simulink model "RPC"  (R2017b)
settings: Solver=FixedStepDiscrete  StartTime=0.0  StopTime=.1  FixedStep=T/100  RelTol=1e-20  AbsTol=1e-20  EnableMultiTasking=on
values from neighbouring files (symbols this model uses):
  n = n(2:3)    [RPC_script.m]
  T = 60/3600/50    (= 0.000333333333333)    [RPC_script.m]    (also in ZPETC_script.m = 0.3)
undefined symbols (not defined in the file or in its folder): d, Wd
libraries: cstblocks x1
settings Model: Creator=oboe  LastModifiedBy=oboe
settings SolverCC: ShapePreserveControl=EnableAll  AutoInsertRateTranBlk=on
settings DataIOCC: LimitDataPoints=on  SaveFormat=Array
settings OptimizationCC: LifeSpan=inf
settings DebuggingCC: SolverPrmCheckMsg=warning  SFUnexpectedBacktrackingDiag=warning  SFNoUnconditionalDefaultTransitionDiag=warning  SFExecutionAtInitializationDiag=none
settings HardwareCC: ProdBitPerPointer=32  ProdBitPerSizeT=32  ProdBitPerPtrDiffT=32  ProdLargestAtomicFloat=None  ProdIntDivRoundTo=Undefined  ProdEndianess=Unspecified  ProdWordSize=32  ProdHWDeviceType=32-bit Generic
settings ModelReferenceCC: PropagateSignalLabelsOutOfModel=off
settings CodeAppCC: StateflowObjectComments=on
settings GRTTargetCC: TargetLangStandard=C89/C90 (ANSI)  GeneratePreprocessorConditionals=Disable all
settings ConfigComp: CovMetricSettings=dw  CovHtmlReporting=on  CovSaveCumulativeToWorkspaceVar=on  CovSaveSingleToWorkspaceVar=on  CovExternalEMLEnable=off  CovSFcnEnable=off

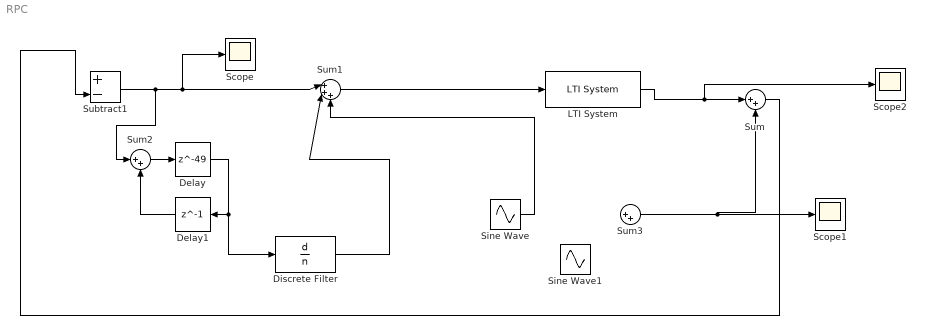
== system RPC ==
  Delay : Delay  DelayLength=49  UseCircularBuffer=on  SampleTime=T
  Delay1 : Delay  DelayLength=1  UseCircularBuffer=on  SampleTime=T
  Discrete Filter : DiscreteFilter  Numerator=d  Denominator=n
  LTI System : cstblocks/LTI System  sys=Wd/(1-Wd)  IC=[]
  Scope : Scope
  Scope1 : Scope
  Scope2 : Scope
  Sine Wave : Sin  Frequency=60.01*2*pi  SampleTime=T
  Sine Wave1 : Sin  Amplitude=.33  Frequency=180*2*pi  Phase=1  SampleTime=T
  Subtract1 : Sum  Inputs=+-
  Sum : Sum  Inputs=|++
  Sum1 : Sum  Inputs=|+++
  Sum2 : Sum  Inputs=|++
  Sum3 : Sum  Inputs=|++
  wires:
  LTI System/1 -> Scope2/1, Sum/1
  Sum/1 -> Subtract1/2
  ? -> Subtract1/1
  Sum1/1 -> LTI System/1
  Sum2/1 -> Delay/1
  Delay1/1 -> Sum2/2
  Delay/1 -> Discrete Filter/1, Delay1/1
  Subtract1/1 -> Sum2/1, Scope/1, Sum1/1
  Discrete Filter/1 -> Sum1/2
  Sum3/1 -> Sum/2, Scope1/1
  Sine Wave/1 -> Sum1/3
